simulink model "hw2_Q2"  (R2022b)
settings: Solver=VariableStepAuto  StartTime=0.0  StopTime=10.0  RelTol=1e-3
settings Model: Creator=shivavafadar  LastModifiedBy=shivavafadar

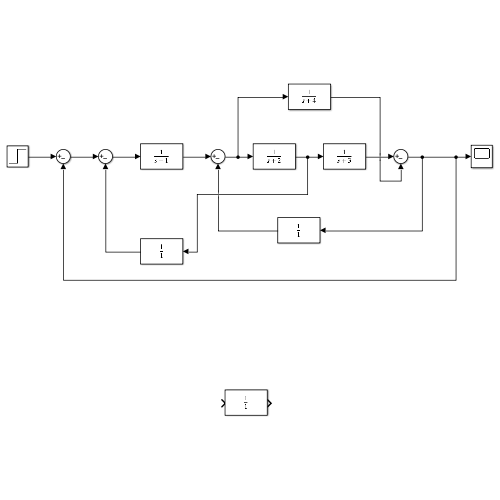
[thumbnail: Simulink's stored preview of the top-level diagram]
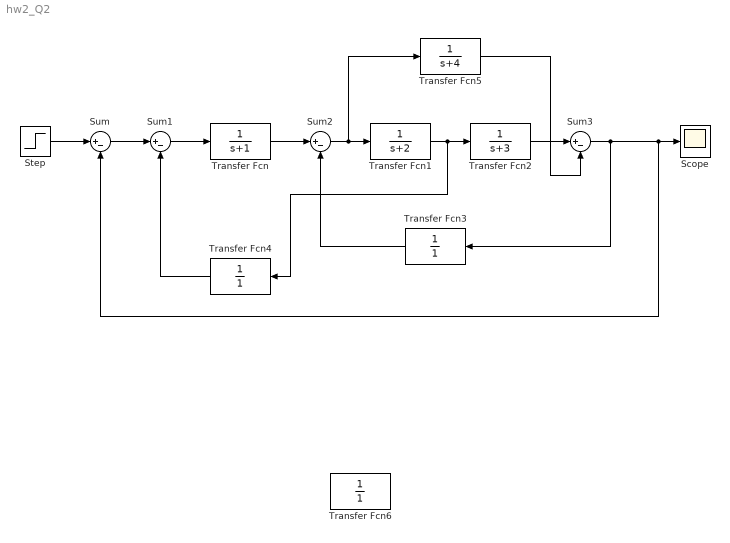
== system hw2_Q2 ==
  Scope : Scope
  Step : Step  SampleTime=0
  Sum{,1..3} (4 alike) : Sum  Inputs=|+-
  Transfer Fcn : TransferFcn  Denominator=[1 1]
  Transfer Fcn1 : TransferFcn  Denominator=[1 2]
  Transfer Fcn2 : TransferFcn  Denominator=[1 3]
  Transfer Fcn3 : TransferFcn  Denominator=[1]
  Transfer Fcn4 : TransferFcn  Denominator=[1]
  Transfer Fcn5 : TransferFcn  Denominator=[1 4]
  Transfer Fcn6 : TransferFcn  Denominator=[1]
  wires:
  Step/1 -> Sum/1
  Sum/1 -> Sum1/1
  Sum1/1 -> Transfer Fcn/1
  Transfer Fcn/1 -> Sum2/1
  Sum2/1 -> Transfer Fcn5/1, Transfer Fcn1/1
  Transfer Fcn1/1 -> Transfer Fcn4/1, Transfer Fcn2/1
  Transfer Fcn2/1 -> Sum3/1
  Sum3/1 -> Scope/1, Sum/2, Transfer Fcn3/1
  Transfer Fcn5/1 -> Sum3/2
  Transfer Fcn3/1 -> Sum2/2
  Transfer Fcn4/1 -> Sum1/2
